simulink model "ej1f"  (R2021a)
settings: Solver=VariableStepAuto  StartTime=0.0  StopTime=30  RelTol=1e-3
values from neighbouring files (symbols this model uses):
  Bm = 2*rand    [codigo.m]
  JL = 10    [codigo.m]
  Jm = 1    [codigo.m]
  KA = 7*(rand+0.5)    [codigo.m]
  KL = 500    [codigo.m]
  Km = 10    [codigo.m]
  Kp = 3    [codigo.m]
  Ra = 1    [codigo.m]
  TL = 5*((5*rand)+1)    [codigo.m]
settings Model: Creator=34622  LastModifiedBy=34622

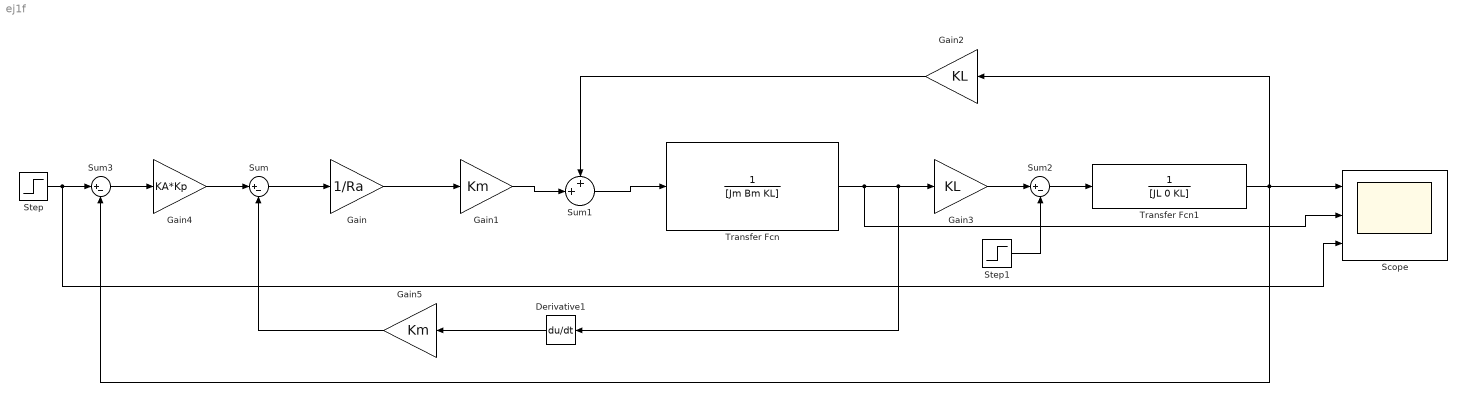
== system ej1f ==
  Derivative1 : Derivative
  Gain : Gain  Gain=1/Ra
  Gain1 : Gain  Gain=Km
  Gain2 : Gain  Gain=KL
  Gain3 : Gain  Gain=KL
  Gain4 : Gain  Gain=KA*Kp
  Gain5 : Gain  Gain=Km
  Scope : Scope  NumInputPorts=3
  Step : Step  Time=0  SampleTime=0
  Step1 : Step  Time=15  After=TL  SampleTime=0
  Sum : Sum  Inputs=|+-
  Sum1 : Sum  Inputs=++|
  Sum2 : Sum  Inputs=|+-
  Sum3 : Sum  Inputs=|+-
  Transfer Fcn : TransferFcn  Denominator=[Jm Bm KL]
  Transfer Fcn1 : TransferFcn  Denominator=[JL 0 KL]
  wires:
  Transfer Fcn/1 -> Scope/2, Derivative1/1, Gain3/1
  Transfer Fcn1/1 -> Gain2/1, Scope/1, Sum3/2
  Derivative1/1 -> Gain5/1
  Sum3/1 -> Gain4/1
  Gain5/1 -> Sum/2
  Step/1 -> Scope/3, Sum3/1
  Sum1/1 -> Transfer Fcn/1
  Gain1/1 -> Sum1/2
  Step1/1 -> Sum2/2
  Sum/1 -> Gain/1
  Gain3/1 -> Sum2/1
  Gain2/1 -> Sum1/1
  Gain4/1 -> Sum/1
  Gain/1 -> Gain1/1
  Sum2/1 -> Transfer Fcn1/1
